simulink model "pitch_rate_simple_model"  (R2024b)
settings: Solver=VariableStepAuto  StartTime=0.0  StopTime=10.0  RelTol=1e-3
libraries: aerolibactuator x1
settings Model: Creator=jonno  LastModifiedBy=jonno

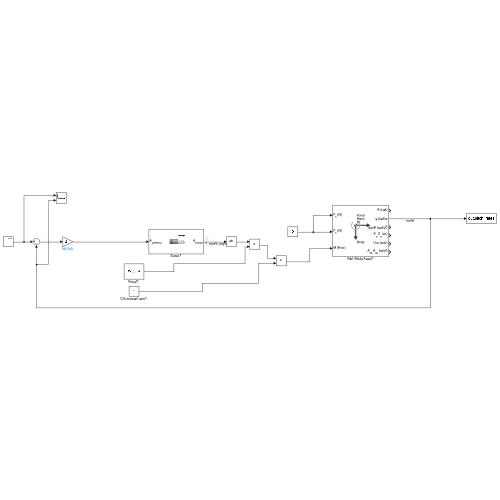
[thumbnail: Simulink's stored preview of the top-level diagram]
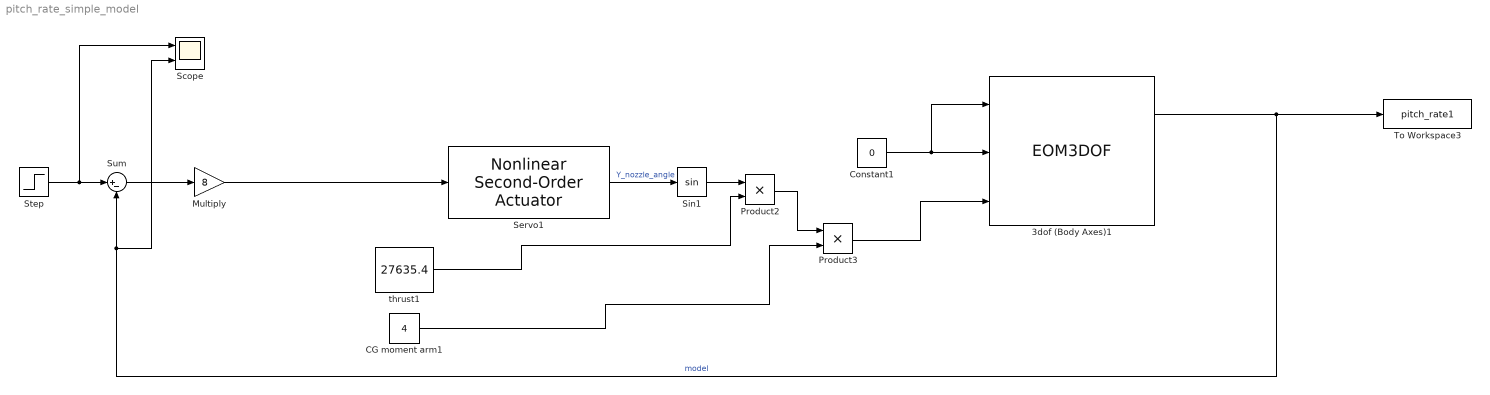
== system pitch_rate_simple_model ==
  3dof (Body Axes)1 : EOM3DOF  v_ini=0  mass=974  Iyy=9470  g=0
  CG moment arm1 : Constant  Value=4
  Constant1 : Constant  Value=0
  Multiply : Gain  Gain=8
  Product2 : Product
  Product3 : Product
  Scope : Scope  NumInputPorts=2
  Servo1 : aerolibactuator/Nonlinear Second-Order Actuator  wn_fin=95  z_fin=0.7  fin_max=10*pi/180  fin_min=-10*pi/180  fin_maxrate=(500*pi/180)  fin_act_0=0  fin_act_vel=0
  Sin1 : Trigonometry
  Step : Step  SampleTime=0
  Sum : Sum  Inputs=|+-
  To Workspace3 : ToWorkspace  VariableName=pitch_rate1  SaveFormat=Timeseries  SampleTime=-1
  thrust1 : Constant  Value=27635.4
  wires:
  Constant1/1 -> 3dof (Body Axes)1/1, 3dof (Body Axes)1/2
  Product2/1 -> Product3/1
  Servo1/1 -> Sin1/1  "Y_nozzle_angle"
  3dof (Body Axes)1/2 -> Scope/2, Sum/2, To Workspace3/1  "model"
  Sin1/1 -> Product2/1
  thrust1/1 -> Product2/2
  CG moment arm1/1 -> Product3/2
  Product3/1 -> 3dof (Body Axes)1/3
  Multiply/1 -> Servo1/1
  Step/1 -> Scope/1, Sum/1
  Sum/1 -> Multiply/1
